simulink model "EA_Quadcopter"  (R2018a)
settings: Solver=VariableStepAuto  StartTime=0.0  StopTime=80  RelTol=1e-3
InitFcn:
  | param
values from neighbouring files (symbols this model uses):
  P = R*P + R2m*[pn;pe;-h]    [animation.m]
undefined symbols (not defined in the file or in its folder): animation, control
settings Model: Creator=mat  LastModifiedBy=mat

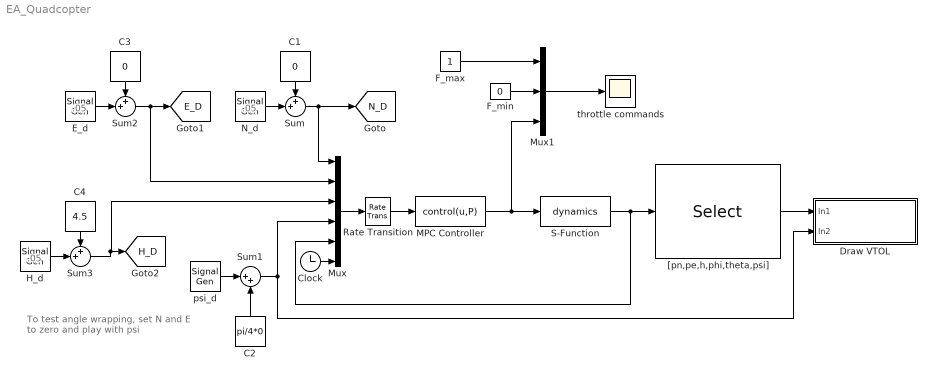
== system EA_Quadcopter ==
  note: .05
  note: .05
  note: .05
  note: To test angle wrapping, set N and E to zero and play with psi
  C1 : Constant  Value=0
  C2 : Constant  Value=pi/4*0
  C3 : Constant  Value=0
  C4 : Constant  Value=4.5
  Clock : Clock
  Draw VTOL : Subsystem
  E_d : SignalGenerator  WaveForm=square  Amplitude=2.5*1  Frequency=.04
  F_max : Constant
  F_min : Constant  Value=0
  H_d : SignalGenerator  WaveForm=square  Amplitude=0.5  Frequency=.01
  MPC Controller : MATLABFcn  MATLABFcn=control(u,P)  OutputDimensions=4
  Mux : Mux  Inputs=6
  Mux1 : Mux  Inputs=3
  N_d : SignalGenerator  WaveForm=square  Amplitude=-2.5*1  Frequency=.02
  Rate Transition : RateTransition  OutPortSampleTime=P.ts*0+.01
  S-Function : S-Function  FunctionName=dynamics  Parameters=P  SFunctionDeploymentMode=off  EnableBusSupport=off
  Sum : Sum  Inputs=++|
  Sum1 : Sum  Inputs=|++
  Sum2 : Sum  Inputs=++|
  Sum3 : Sum  Inputs=++|
  "[pn,pe,h,phi,theta,psi]" : Selector  InputPortWidth=12  IndexOptions=Index vector (dialog)  Indices=[1 2 3 4 5 6]  OutputSizes=1
  psi_d : SignalGenerator  WaveForm=square  Amplitude=pi/4*1  Frequency=.03
  throttle commands : Scope
  tag scope: E_D=global, H_D=global, N_D=global
  wires:
  C1/1 -> Sum/1
  MPC Controller/1 -> Mux1/3, S-Function/1
  F_max/1 -> Mux1/1
  "[pn,pe,h,phi,theta,psi]"/1 -> Draw VTOL/1(In1)
  Mux/1 -> Rate Transition/1
  F_min/1 -> Mux1/2
  psi_d/1 -> Sum1/1
  C2/1 -> Sum1/2
  S-Function/1 -> Mux/5, "[pn,pe,h,phi,theta,psi]"/1
  Rate Transition/1 -> MPC Controller/1
  Sum/1 -> Mux/1, [N_D]
  Sum1/1 -> Mux/4, Draw VTOL/2(In2)
  N_d/1 -> Sum/2
  Mux1/1 -> throttle commands/1
  Clock/1 -> Mux/6
  E_d/1 -> Sum2/2
  C3/1 -> Sum2/1
  Sum2/1 -> Mux/2, [E_D]
  H_d/1 -> Sum3/2
  C4/1 -> Sum3/1
  Sum3/1 -> Mux/3, [H_D]

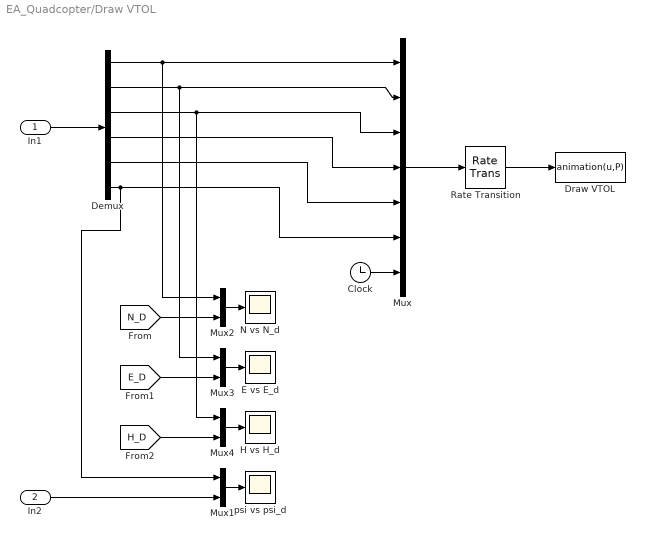
== system EA_Quadcopter/Draw VTOL ==
  In1 : Inport
  In2 : Inport  Port=2
  Clock : Clock
  Demux : Demux  Outputs=6
  Draw VTOL : MATLABFcn  MATLABFcn=animation(u,P)  OutputDimensions=0
  E vs E_d : Scope
  H vs H_d : Scope
  Mux : Mux  Inputs=7
  Mux{1..4} (4 alike) : Mux  Inputs=2
  N vs N_d : Scope
  Rate Transition : RateTransition  OutPortSampleTime=P.t_plot
  psi vs psi_d : Scope
  wires:
  In1/1 -> Demux/1
  Demux/1 -> Mux2/1, Mux/1
  Demux/2 -> Mux3/1, Mux/2
  Rate Transition/1 -> Draw VTOL/1
  Mux/1 -> Rate Transition/1
  In2/1 -> Mux1/2
  Mux1/1 -> psi vs psi_d/1
  Mux2/1 -> N vs N_d/1
  [N_D] -> Mux2/2
  Demux/3 -> Mux4/1, Mux/3
  Demux/4 -> Mux/4
  Clock/1 -> Mux/7
  Demux/5 -> Mux/5
  Demux/6 -> Mux1/1, Mux/6
  Mux3/1 -> E vs E_d/1
  Mux4/1 -> H vs H_d/1
  [E_D] -> Mux3/2
  [H_D] -> Mux4/2
